simulink model "BMS"  (R2025b)
settings: Solver=VariableStepAuto  StartTime=0.0  StopTime=100000  RelTol=1e-3
libraries: fl_lib x15, nesl_utility x15, ee_lib x6, batteryecm_lib x5
settings DebuggingCC: AlgebraicLoopMsg=none

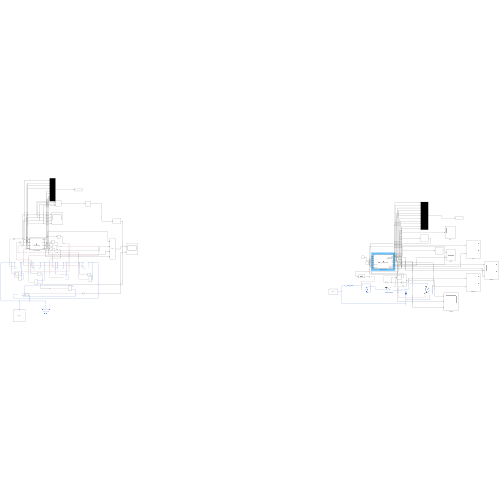
[thumbnail: Simulink's stored preview of the top-level diagram]
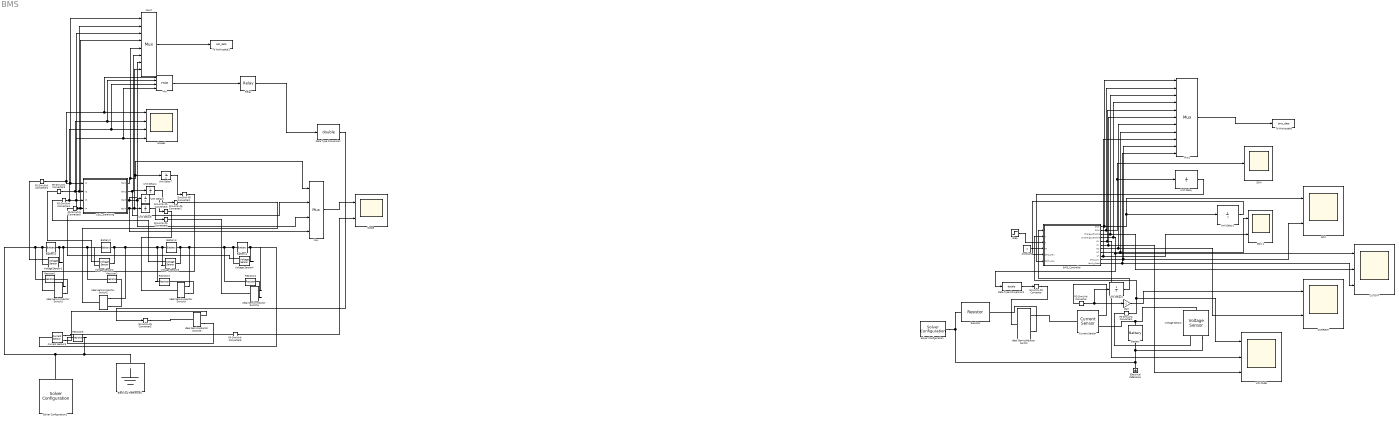
== system BMS ==
  BMS_Controller : MATLAB Function  TreatAsAtomicUnit=on
  Battery : batteryecm_lib/Battery  Vnom=48 V  prm_dir=simscape.enum.battery.prm_dir.disabled  R1_dis=2 Ohm  R1_ch=2 Ohm  R1=0.02 Ohm  prm_AH=simscape.enum.battery.prm_AH.finite  AH=50 A*hr  V1=46 V  AH1=40 A*hr  prm_R2=simscape.enum.battery.prm_R2.disabled  R2=2000 Ohm  Tmeas=298.15 K  charge_measurement_port=simscape.enum.battery.enable.no  prm_dyn=simscape.enum.battery.prm_dyn.off  Rp1=0.005 Ohm  tau1=30 s  Rp2=0.005 Ohm  tau2=30 s  Rp3=0.005 Ohm  tau3=30 s  Rp4=0.005 Ohm  tau4=30 s  Rp5=0.005 Ohm  tau5=30 s  prm_fade=simscape.enum.battery.prm_fade.disabled  N_fade=100  AH_fade=45 A*hr  R1_fade=2.02 Ohm  R1_ch_fade=2.02 Ohm  V1_fade=10.35 V  prm_age=simscape.enum.battery.prm_age.disabled  prm_age_OCV=simscape.enum.battery.prm_age_OCV.OCV  OCV_age=0.9  SOC_age=60  Tmeas_age=298.15 K  delta_time_age_vec=[0] d  temperature_age_vec=[273] K  OCV_scaling_age=2.2134e6  OCV_offset_age=1.632e6  temp_exp_age=0.515833569 V  t_exp_age=0.75  Vnom_T2=12 V  R1_T2=2.2 Ohm  R1_T2_dis=2.2 Ohm  R1_T2_ch=2.2 Ohm  V1_T2=11.4 V  R2_T2=2200 Ohm  Rp1_T2=0.005 Ohm  tau1_T2=30 s  Rp2_T2=0.005 Ohm  tau2_T2=30 s  Rp3_T2=0.005 Ohm  tau3_T2=30 s  Rp4_T2=0.005 Ohm  tau4_T2=30 s  Rp5_T2=0.005 Ohm  tau5_T2=30 s  Tmeas2=273.15 K  thermal_port=simscape.enum.thermaleffects.omit  thermal_mass=30000 J/K  i_specify=off  i_priority=None  i=0 A  i_nominal_specify=off  i_nominal_value=1  i_nominal_unit=A  v_specify=off  v_priority=None  v=0 V  v_nominal_specify=off  v_nominal_value=1  v_nominal_unit=V  charge_specify=off  charge_priority=High  charge=50 A*hr  charge_nominal_specify=off  charge_nominal_value=1  charge_nominal_unit=A*hr  num_cycles_specify=off  num_cycles_priority=High  num_cycles=0  num_cycles_nominal_specify=off  num_cycles_nominal_value=1  num_cycles_nominal_unit=1  temperature_specify=off  temperature_priority=High  temperature=298.15 K  temperature_nominal_specify=off  temperature_nominal_value=1  temperature_nominal_unit=K
  Battery1 : batteryecm_lib/Battery  Vnom=3.7 V  prm_dir=simscape.enum.battery.prm_dir.disabled  R1_dis=2 Ohm  R1_ch=2 Ohm  R1=0.02 Ohm  prm_AH=simscape.enum.battery.prm_AH.finite  AH=3 Ah  V1=3.45 V  AH1=2.7 Ah  prm_R2=simscape.enum.battery.prm_R2.disabled  R2=2000 Ohm  Tmeas=298.15 K  charge_measurement_port=simscape.enum.battery.enable.no  prm_dyn=simscape.enum.battery.prm_dyn.off  Rp1=0.005 Ohm  tau1=30 s  Rp2=0.005 Ohm  tau2=30 s  Rp3=0.005 Ohm  tau3=30 s  Rp4=0.005 Ohm  tau4=30 s  Rp5=0.005 Ohm  tau5=30 s  prm_fade=simscape.enum.battery.prm_fade.disabled  N_fade=100  AH_fade=45 A*hr  R1_fade=2.02 Ohm  R1_ch_fade=2.02 Ohm  V1_fade=10.35 V  prm_age=simscape.enum.battery.prm_age.disabled  prm_age_OCV=simscape.enum.battery.prm_age_OCV.OCV  OCV_age=0.9  SOC_age=60  Tmeas_age=298.15 K  delta_time_age_vec=[0] d  temperature_age_vec=[273] K  OCV_scaling_age=2.2134e6  OCV_offset_age=1.632e6  temp_exp_age=0.515833569 V  t_exp_age=0.75  Vnom_T2=12 V  R1_T2=2.2 Ohm  R1_T2_dis=2.2 Ohm  R1_T2_ch=2.2 Ohm  V1_T2=11.4 V  R2_T2=2200 Ohm  Rp1_T2=0.005 Ohm  tau1_T2=30 s  Rp2_T2=0.005 Ohm  tau2_T2=30 s  Rp3_T2=0.005 Ohm  tau3_T2=30 s  Rp4_T2=0.005 Ohm  tau4_T2=30 s  Rp5_T2=0.005 Ohm  tau5_T2=30 s  Tmeas2=273.15 K  thermal_port=simscape.enum.thermaleffects.omit  thermal_mass=30000 J/K  i_specify=off  i_priority=None  i=0 A  i_nominal_specify=off  i_nominal_value=1  i_nominal_unit=A  v_specify=off  v_priority=None  v=0 V  v_nominal_specify=off  v_nominal_value=1  v_nominal_unit=V  charge_specify=on  charge_priority=High  charge=2.7 Ah  charge_nominal_specify=off  charge_nominal_value=1  charge_nominal_unit=A*hr  num_cycles_specify=off  num_cycles_priority=High  num_cycles=0  num_cycles_nominal_specify=off  num_cycles_nominal_value=1  num_cycles_nominal_unit=1  temperature_specify=off  temperature_priority=High  temperature=298.15 K  temperature_nominal_specify=off  temperature_nominal_value=1  temperature_nominal_unit=K
  Battery2 : batteryecm_lib/Battery  Vnom=3.7 V  prm_dir=simscape.enum.battery.prm_dir.disabled  R1_dis=2 Ohm  R1_ch=2 Ohm  R1=0.02 Ohm  prm_AH=simscape.enum.battery.prm_AH.finite  AH=3 Ah  V1=3.35 V  AH1=2.4 Ah  prm_R2=simscape.enum.battery.prm_R2.disabled  R2=2000 Ohm  Tmeas=298.15 K  charge_measurement_port=simscape.enum.battery.enable.no  prm_dyn=simscape.enum.battery.prm_dyn.off  Rp1=0.005 Ohm  tau1=30 s  Rp2=0.005 Ohm  tau2=30 s  Rp3=0.005 Ohm  tau3=30 s  Rp4=0.005 Ohm  tau4=30 s  Rp5=0.005 Ohm  tau5=30 s  prm_fade=simscape.enum.battery.prm_fade.disabled  N_fade=100  AH_fade=45 A*hr  R1_fade=2.02 Ohm  R1_ch_fade=2.02 Ohm  V1_fade=10.35 V  prm_age=simscape.enum.battery.prm_age.disabled  prm_age_OCV=simscape.enum.battery.prm_age_OCV.OCV  OCV_age=0.9  SOC_age=60  Tmeas_age=298.15 K  delta_time_age_vec=[0] d  temperature_age_vec=[273] K  OCV_scaling_age=2.2134e6  OCV_offset_age=1.632e6  temp_exp_age=0.515833569 V  t_exp_age=0.75  Vnom_T2=12 V  R1_T2=2.2 Ohm  R1_T2_dis=2.2 Ohm  R1_T2_ch=2.2 Ohm  V1_T2=11.4 V  R2_T2=2200 Ohm  Rp1_T2=0.005 Ohm  tau1_T2=30 s  Rp2_T2=0.005 Ohm  tau2_T2=30 s  Rp3_T2=0.005 Ohm  tau3_T2=30 s  Rp4_T2=0.005 Ohm  tau4_T2=30 s  Rp5_T2=0.005 Ohm  tau5_T2=30 s  Tmeas2=273.15 K  thermal_port=simscape.enum.thermaleffects.omit  thermal_mass=30000 J/K  i_specify=off  i_priority=None  i=0 A  i_nominal_specify=off  i_nominal_value=1  i_nominal_unit=A  v_specify=off  v_priority=None  v=0 V  v_nominal_specify=off  v_nominal_value=1  v_nominal_unit=V  charge_specify=on  charge_priority=High  charge=2.4 Ah  charge_nominal_specify=off  charge_nominal_value=1  charge_nominal_unit=A*hr  num_cycles_specify=off  num_cycles_priority=High  num_cycles=0  num_cycles_nominal_specify=off  num_cycles_nominal_value=1  num_cycles_nominal_unit=1  temperature_specify=off  temperature_priority=High  temperature=298.15 K  temperature_nominal_specify=off  temperature_nominal_value=1  temperature_nominal_unit=K
  Battery3 : batteryecm_lib/Battery  Vnom=3.7 V  prm_dir=simscape.enum.battery.prm_dir.disabled  R1_dis=2 Ohm  R1_ch=2 Ohm  R1=0.02 Ohm  prm_AH=simscape.enum.battery.prm_AH.finite  AH=3 Ah  V1=3.25 V  AH1=2.1 Ah  prm_R2=simscape.enum.battery.prm_R2.disabled  R2=2000 Ohm  Tmeas=298.15 K  charge_measurement_port=simscape.enum.battery.enable.no  prm_dyn=simscape.enum.battery.prm_dyn.off  Rp1=0.005 Ohm  tau1=30 s  Rp2=0.005 Ohm  tau2=30 s  Rp3=0.005 Ohm  tau3=30 s  Rp4=0.005 Ohm  tau4=30 s  Rp5=0.005 Ohm  tau5=30 s  prm_fade=simscape.enum.battery.prm_fade.disabled  N_fade=100  AH_fade=45 A*hr  R1_fade=2.02 Ohm  R1_ch_fade=2.02 Ohm  V1_fade=10.35 V  prm_age=simscape.enum.battery.prm_age.disabled  prm_age_OCV=simscape.enum.battery.prm_age_OCV.OCV  OCV_age=0.9  SOC_age=60  Tmeas_age=298.15 K  delta_time_age_vec=[0] d  temperature_age_vec=[273] K  OCV_scaling_age=2.2134e6  OCV_offset_age=1.632e6  temp_exp_age=0.515833569 V  t_exp_age=0.75  Vnom_T2=12 V  R1_T2=2.2 Ohm  R1_T2_dis=2.2 Ohm  R1_T2_ch=2.2 Ohm  V1_T2=11.4 V  R2_T2=2200 Ohm  Rp1_T2=0.005 Ohm  tau1_T2=30 s  Rp2_T2=0.005 Ohm  tau2_T2=30 s  Rp3_T2=0.005 Ohm  tau3_T2=30 s  Rp4_T2=0.005 Ohm  tau4_T2=30 s  Rp5_T2=0.005 Ohm  tau5_T2=30 s  Tmeas2=273.15 K  thermal_port=simscape.enum.thermaleffects.omit  thermal_mass=30000 J/K  i_specify=off  i_priority=None  i=0 A  i_nominal_specify=off  i_nominal_value=1  i_nominal_unit=A  v_specify=off  v_priority=None  v=0 V  v_nominal_specify=off  v_nominal_value=1  v_nominal_unit=V  charge_specify=on  charge_priority=High  charge=2.1 Ah  charge_nominal_specify=off  charge_nominal_value=1  charge_nominal_unit=A*hr  num_cycles_specify=off  num_cycles_priority=High  num_cycles=0  num_cycles_nominal_specify=off  num_cycles_nominal_value=1  num_cycles_nominal_unit=1  temperature_specify=off  temperature_priority=High  temperature=298.15 K  temperature_nominal_specify=off  temperature_nominal_value=1  temperature_nominal_unit=K
  Battery4 : batteryecm_lib/Battery  Vnom=3.7 V  prm_dir=simscape.enum.battery.prm_dir.disabled  R1_dis=2 Ohm  R1_ch=2 Ohm  R1=0.02 Ohm  prm_AH=simscape.enum.battery.prm_AH.finite  AH=3 Ah  V1=3.15 V  AH1=1.8 Ah  prm_R2=simscape.enum.battery.prm_R2.disabled  R2=2000 Ohm  Tmeas=298.15 K  charge_measurement_port=simscape.enum.battery.enable.no  prm_dyn=simscape.enum.battery.prm_dyn.off  Rp1=0.005 Ohm  tau1=30 s  Rp2=0.005 Ohm  tau2=30 s  Rp3=0.005 Ohm  tau3=30 s  Rp4=0.005 Ohm  tau4=30 s  Rp5=0.005 Ohm  tau5=30 s  prm_fade=simscape.enum.battery.prm_fade.disabled  N_fade=100  AH_fade=45 A*hr  R1_fade=2.02 Ohm  R1_ch_fade=2.02 Ohm  V1_fade=10.35 V  prm_age=simscape.enum.battery.prm_age.disabled  prm_age_OCV=simscape.enum.battery.prm_age_OCV.OCV  OCV_age=0.9  SOC_age=60  Tmeas_age=298.15 K  delta_time_age_vec=[0] d  temperature_age_vec=[273] K  OCV_scaling_age=2.2134e6  OCV_offset_age=1.632e6  temp_exp_age=0.515833569 V  t_exp_age=0.75  Vnom_T2=12 V  R1_T2=2.2 Ohm  R1_T2_dis=2.2 Ohm  R1_T2_ch=2.2 Ohm  V1_T2=11.4 V  R2_T2=2200 Ohm  Rp1_T2=0.005 Ohm  tau1_T2=30 s  Rp2_T2=0.005 Ohm  tau2_T2=30 s  Rp3_T2=0.005 Ohm  tau3_T2=30 s  Rp4_T2=0.005 Ohm  tau4_T2=30 s  Rp5_T2=0.005 Ohm  tau5_T2=30 s  Tmeas2=273.15 K  thermal_port=simscape.enum.thermaleffects.omit  thermal_mass=30000 J/K  i_specify=off  i_priority=None  i=0 A  i_nominal_specify=off  i_nominal_value=1  i_nominal_unit=A  v_specify=off  v_priority=None  v=0 V  v_nominal_specify=off  v_nominal_value=1  v_nominal_unit=V  charge_specify=on  charge_priority=High  charge=1.8 Ah  charge_nominal_specify=off  charge_nominal_value=1  charge_nominal_unit=A*hr  num_cycles_specify=off  num_cycles_priority=High  num_cycles=0  num_cycles_nominal_specify=off  num_cycles_nominal_value=1  num_cycles_nominal_unit=1  temperature_specify=off  temperature_priority=High  temperature=298.15 K  temperature_nominal_specify=off  temperature_nominal_value=1  temperature_nominal_unit=K
  CELL_Balancing : MATLAB Function  TreatAsAtomicUnit=on
  CURRENT : Scope  NumInputPorts=2
      settings: ActiveDisplayYMinimum=-24.113371295047806  ActiveDisplayYMaximum=65.015748640986715
  CUTOFF : Scope  NumInputPorts=3
      settings: ActiveDisplayString=3  ActiveDisplayYMinimum=-1  ActiveDisplayYMaximum=7  DataLoggingVariableName=ScopeData2
  Constant : Constant
  Current Sensor : fl_lib/Electrical/Electrical Sensors/Current Sensor
  Current Sensor3 : fl_lib/Electrical/Electrical Sensors/Current Sensor
  Data Type Conversion : DataTypeConversion  OutDataTypeStr=double  SaturateOnIntegerOverflow=off  RndMeth=Floor
  Data Type Conversion1 : DataTypeConversion  OutDataTypeStr=double  SaturateOnIntegerOverflow=off  RndMeth=Floor
  Electrical Reference : fl_lib/Electrical/Electrical Elements/Electrical Reference
  Electrical Reference1 : fl_lib/Electrical/Electrical Elements/Electrical Reference
  Gain : Gain  Gain=-1
  Ideal Semiconductor Switch : ee_lib/Semiconductors & Converters/Ideal Semiconductor Switch  port_option=ee.enum.controlport.ps  Ron=0.001 Ohm  Goff=1e-6 1/Ohm  Vth=0.5 V  diode_param=ee.enum.semiconductors.protectionDiode.nodynamics  diode_Vf=0.8 V  diode_Ron=0.001 Ohm  diode_Goff=1e-5 1/Ohm  diode_C=50e-9 F  diode_iRM=-235 A  diode_iF=300 A  diode_idot=-50 A/us  diode_trr_param=ee.enum.converters.diodetrr.trr_factor  diode_trr_factor=3  diode_trr=15 us  diode_Qrr=1500 s*uA
  Ideal Semiconductor Switch{1..5} (5 alike) : ee_lib/Semiconductors & Converters/Ideal Semiconductor Switch  port_option=ee.enum.controlport.ps  Ron=0.1 Ohm  Goff=1e-6 S  Vth=0.5 V  diode_param=ee.enum.semiconductors.protectionDiode.external  diode_Vf=0.8 V  diode_Ron=0.001 Ohm  diode_Goff=1e-5 1/Ohm  diode_C=50e-9 F  diode_iRM=-235 A  diode_iF=300 A  diode_idot=-50 A/us  diode_trr_param=ee.enum.converters.diodetrr.trr_factor  diode_trr_factor=3  diode_trr=15 us  diode_Qrr=1500 s*uA
  Min : MinMax  Inputs=4
  Mux : Mux
  Mux1 : Mux  Inputs=11
  Mux2 : Mux  Inputs=8
  PS-Simulink Converter{,1..6} (7 alike) : nesl_utility/PS-Simulink Converter  PhysicalDomain=network_engine_domain  SubClassName=ps_output  LeftPortType=input  RightPortType=output  PseudoPeriodic=off  Frequencies=[]  VectorFormat=inherit  Unit=inherit  AffineConversion=off
  Relay : Relay  OnSwitchValue=3.0  OffSwitchValue=2.8
  Resistor : fl_lib/Electrical/Electrical Elements/Resistor  R=10 Ohm  i_specify=off  i_priority=None  i=0 A  i_nominal_specify=off  i_nominal_value=1  i_nominal_unit=A  v_specify=off  v_priority=None  v=0 V  v_nominal_specify=off  v_nominal_value=1  v_nominal_unit=V
  Resistor{1..4} (4 alike) : fl_lib/Electrical/Electrical Elements/Resistor  R=100 Ohm  i_specify=off  i_priority=None  i=0 A  i_nominal_specify=off  i_nominal_value=1  i_nominal_unit=A  v_specify=off  v_priority=None  v=0 V  v_nominal_specify=off  v_nominal_value=1  v_nominal_unit=V
  Resistor5 : fl_lib/Electrical/Electrical Elements/Resistor  R=50 Ohm  i_specify=off  i_priority=None  i=0 A  i_nominal_specify=off  i_nominal_value=1  i_nominal_unit=A  v_specify=off  v_priority=None  v=0 V  v_nominal_specify=off  v_nominal_value=1  v_nominal_unit=V
  "SOC " : Scope  NumInputPorts=2
      settings: ActiveDisplayYMinimum=0  ActiveDisplayYMaximum=1.05
  SOC 1 : Scope  NumInputPorts=2
      settings: ActiveDisplayYMinimum=-1  ActiveDisplayYMaximum=2  DataLoggingVariableName=ScopeData7
  SOH : Scope
      settings: ActiveDisplayYMinimum=0.7  ActiveDisplayYMaximum=1.01  DataLoggingVariableName=ScopeData4
  Scope : Scope  NumInputPorts=2
      settings: ActiveDisplayYMinimum=-0.08125912986411854  ActiveDisplayYMaximum=1.0773261926772566  DataLoggingVariableName=ScopeData5
  Scope1 : Scope  NumInputPorts=4
      settings: ActiveDisplayString=4  ActiveDisplayYMinimum=2  ActiveDisplayYMaximum=5  DataLoggingVariableName=ScopeData6
  Simulink-PS Converter{,1..5} (6 alike) : nesl_utility/Simulink-PS Converter  PhysicalDomain=network_engine_domain  SubClassName=ps_input  LeftPortType=input  RightPortType=output  PseudoPeriodic=off  Frequencies=[]  NoiseDistribution=none  NoiseParameters=[]  Unit=1  AffineConversion=off  FilteringAndDerivatives=provide  SimscapeFilterOrder=1  InputFilterTimeConstant=0.001  UdotUserProvided=0
  Solver Configuration : nesl_utility/Solver Configuration  PhysicalDomain=network_engine_domain  SubClassName=solver  LeftPortType=input  RightPortType=generic  Tones=[]  Harmonics=[]  SimulateNoise=off  Profile=off  UseLocalSampling=off  EnableSwitchedLinearOptims=on  FrequencyDomain=off  UseCCode=off  RelTol=0.001  AbsTol=0.001  MinStep=1e-09  ToWorkspace=off  RevertToSquareIcSolve=off  NumHomotopyIterations=100  PhasorMode=off  PhasorModeNumHarmonics=1  ConsistencySolver=NEWTON_XTOL_AFTER_FTOL  IndexReductionMethod=DerivativeReplacement  DoDC=off  ResidualTolerance=1e-09  ConsistencyTolSource=GLOBAL  ConsistencyAbsTol=0.001  ConsistencyRelTol=0.001  ConsistencyTolFactor=0.001  UseLocalSolver=off  LocalSolverChoice=NE_BACKWARD_EULER_ADVANCER  ResolveIndetEquations=on  FunctionEvalNumThread=1  LocalSolverSampleTime=0.001  DoFixedCost=off  MaxNonlinIter=3  MaxModeIter=2  ComputeImpulses=off  ImpulseIterations=2  LinearAlgebra=auto  LinearAlgebraNumThread=0  EquationFormulation=NE_TIME_EF  DelaysMemoryBudget=1024  AutomaticFiltering=on  FilteringTimeConstant=0.001  PartitionStorageMethod=AS_NEEDED  PartitionMemoryBudget=1024  PartitionMethod=ROBUST  MultibodyUseLocalSolver=off  MultibodyLocalSolverChoice=ODE1  MultibodyLocalSolverSampleTime=0.001
  Solver Configuration1 : nesl_utility/Solver Configuration  PhysicalDomain=network_engine_domain  SubClassName=solver  LeftPortType=input  RightPortType=generic  Tones=[]  Harmonics=[]  SimulateNoise=off  Profile=off  UseLocalSampling=off  EnableSwitchedLinearOptims=on  FrequencyDomain=off  UseCCode=off  RelTol=0.001  AbsTol=0.001  MinStep=1e-09  ToWorkspace=off  RevertToSquareIcSolve=off  NumHomotopyIterations=100  PhasorMode=off  PhasorModeNumHarmonics=1  ConsistencySolver=NEWTON_XTOL_AFTER_FTOL  IndexReductionMethod=DerivativeReplacement  DoDC=off  ResidualTolerance=1e-09  ConsistencyTolSource=GLOBAL  ConsistencyAbsTol=0.001  ConsistencyRelTol=0.001  ConsistencyTolFactor=0.001  UseLocalSolver=off  LocalSolverChoice=NE_BACKWARD_EULER_ADVANCER  ResolveIndetEquations=on  FunctionEvalNumThread=1  LocalSolverSampleTime=0.001  DoFixedCost=off  MaxNonlinIter=3  MaxModeIter=2  ComputeImpulses=off  ImpulseIterations=2  LinearAlgebra=auto  LinearAlgebraNumThread=0  EquationFormulation=NE_TIME_EF  DelaysMemoryBudget=1024  AutomaticFiltering=on  FilteringTimeConstant=0.001  PartitionStorageMethod=AS_NEEDED  PartitionMemoryBudget=1024  PartitionMethod=ROBUST  MultibodyUseLocalSolver=off  MultibodyLocalSolverChoice=ODE1  MultibodyLocalSolverSampleTime=0.001
  Step : Step  Time=5000  Before=25  After=70  SampleTime=0
  To Workspace : ToWorkspace  VariableName=bms_data  SaveFormat=Structure With Time  SampleTime=-1
  To Workspace1 : ToWorkspace  VariableName=cell_data  SaveFormat=Structure With Time  SampleTime=-1
  Unit Delay : UnitDelay  InitialCondition=1  HasFrameUpgradeWarning=on
  Unit Delay1 : UnitDelay  InitialCondition=1  HasFrameUpgradeWarning=on
  Unit Delay2 : UnitDelay  HasFrameUpgradeWarning=on
  Unit Delay{4..7} (4 alike) : UnitDelay  SampleTime=-1  HasFrameUpgradeWarning=on
  VOLTAGE : Scope  NumInputPorts=3
      settings: ActiveDisplayString=3  ActiveDisplayYMinimum=-5  ActiveDisplayYMaximum=54  DataLoggingVariableName=ScopeData3
  Voltage Sensor{,1..4} (5 alike) : fl_lib/Electrical/Electrical Sensors/Voltage Sensor
  wires:
  PS-Simulink Converter/1 -> Unit Delay2/1, Gain/1
  PS-Simulink Converter1/1 -> BMS_Controller/2(V), VOLTAGE/1
  Constant/1 -> BMS_Controller/4(Ts)
  BMS_Controller/1(SOC) -> Mux1/1, "SOC "/1, Unit Delay1/1
  Unit Delay1/1 -> BMS_Controller/5(SOC_prev)
  Gain/1 -> CURRENT/1
  BMS_Controller/5(OV) -> Mux1/5, VOLTAGE/2
  BMS_Controller/2(SOH) -> Mux1/2, SOH/1, Unit Delay/1
  Unit Delay2/1 -> BMS_Controller/1(I)
  PS-Simulink Converter2/1 -> Min/1, Scope1/1, Mux2/1, CELL_Balancing/1(V1)
  PS-Simulink Converter3/1 -> Min/2, Scope1/2, CELL_Balancing/2(V2), Mux2/2
  PS-Simulink Converter4/1 -> Mux2/3, CELL_Balancing/3(V3), Min/3, Scope1/3
  CELL_Balancing/1(Bal1) -> Mux2/5, Unit Delay7/1, Mux/1
  CELL_Balancing/2(Bal2) -> Mux2/6, Unit Delay4/1, Mux/2
  CELL_Balancing/3(Bal3) -> Mux2/7, Unit Delay5/1, Mux/3
  Unit Delay7/1 -> Simulink-PS Converter1/1
  Unit Delay4/1 -> Simulink-PS Converter2/1
  Unit Delay5/1 -> Simulink-PS Converter3/1
  Unit Delay6/1 -> Simulink-PS Converter4/1
  Mux/1 -> Scope/1
  PS-Simulink Converter6/1 -> Scope/2
  Data Type Conversion/1 -> Simulink-PS Converter5/1
  CELL_Balancing/4(Bal4) -> Mux/4, Mux2/8, Unit Delay6/1
  Min/1 -> Relay/1
  Relay/1 -> Data Type Conversion/1
  Unit Delay/1 -> BMS_Controller/6(SOH_prev)
  Step/1 -> BMS_Controller/3(T)
  BMS_Controller/7(OC) -> Mux1/7, CURRENT/2
  BMS_Controller/10(SOC_Low) -> Mux1/10, "SOC "/2
  BMS_Controller/8(OT) -> Mux1/8, SOC 1/1
  BMS_Controller/9(UT) -> Mux1/9, SOC 1/2
  BMS_Controller/6(UV) -> Mux1/6, VOLTAGE/3
  BMS_Controller/4(Discharge_Enable) -> Mux1/4, Data Type Conversion1/1, CUTOFF/1
  Data Type Conversion1/1 -> Simulink-PS Converter/1
  BMS_Controller/3(Charge_Enable) -> Mux1/3, CUTOFF/2
  BMS_Controller/11(Fault_Code) -> Mux1/11, CUTOFF/3
  Mux1/1 -> To Workspace/1
  PS-Simulink Converter5/1 -> Mux2/4, CELL_Balancing/4(V4), Min/4, Scope1/4
  Mux2/1 -> To Workspace1/1
  connections:
  Battery/RConn1 -- Voltage Sensor/RConn2 -- Electrical Reference/LConn1 -- Solver Configuration/RConn1 -- Resistor/LConn1
  Battery/LConn1 -- Current Sensor/RConn2 -- Voltage Sensor/LConn1
  PS-Simulink Converter/LConn1 -- Current Sensor/RConn1
  PS-Simulink Converter1/LConn1 -- Voltage Sensor/RConn1
  Current Sensor/LConn1 -- Ideal Semiconductor Switch/RConn1
  Simulink-PS Converter/RConn1 -- Ideal Semiconductor Switch/LConn1
  Ideal Semiconductor Switch/RConn2 -- Resistor/RConn1
  PS-Simulink Converter2/LConn1 -- Voltage Sensor1/RConn1
  Voltage Sensor4/LConn1 -- Current Sensor3/LConn1 -- Ideal Semiconductor Switch4/RConn1 -- Battery4/LConn1
  PS-Simulink Converter5/LConn1 -- Voltage Sensor4/RConn1
  PS-Simulink Converter3/LConn1 -- Voltage Sensor2/RConn1
  PS-Simulink Converter4/LConn1 -- Voltage Sensor3/RConn1
  Ideal Semiconductor Switch1/RConn2 -- Resistor1/LConn1
  Ideal Semiconductor Switch2/RConn2 -- Resistor2/LConn1
  Ideal Semiconductor Switch3/RConn2 -- Resistor3/LConn1
  Ideal Semiconductor Switch4/RConn2 -- Resistor4/LConn1
  Simulink-PS Converter2/RConn1 -- Ideal Semiconductor Switch2/LConn1
  Simulink-PS Converter3/RConn1 -- Ideal Semiconductor Switch3/LConn1
  Simulink-PS Converter4/RConn1 -- Ideal Semiconductor Switch4/LConn1
  Voltage Sensor1/LConn1 -- Resistor2/RConn1 -- Voltage Sensor2/RConn2 -- Battery2/RConn1 -- Ideal Semiconductor Switch1/RConn1 -- Battery1/LConn1
  Voltage Sensor2/LConn1 -- Resistor3/RConn1 -- Voltage Sensor3/RConn2 -- Battery3/RConn1 -- Ideal Semiconductor Switch2/RConn1 -- Battery2/LConn1
  Voltage Sensor3/LConn1 -- Voltage Sensor4/RConn2 -- Battery4/RConn1 -- Resistor4/RConn1 -- Ideal Semiconductor Switch3/RConn1 -- Battery3/LConn1
  Current Sensor3/RConn1 -- PS-Simulink Converter6/LConn1
  Current Sensor3/RConn2 -- Ideal Semiconductor Switch5/RConn1
  Ideal Semiconductor Switch5/RConn2 -- Resistor5/LConn1
  Simulink-PS Converter5/RConn1 -- Ideal Semiconductor Switch5/LConn1
  Simulink-PS Converter1/RConn1 -- Ideal Semiconductor Switch1/LConn1
  Battery1/RConn1 -- Voltage Sensor1/RConn2 -- Resistor1/RConn1 -- Resistor5/RConn1 -- Electrical Reference1/LConn1 -- Solver Configuration1/RConn1

== matlab function BMS/CELL_Balancing ==
  data: V1 input; Bal1 output; V2 input; V3 input; V4 input; Bal2 output; Bal3 output; Bal4 output
function [Bal1, Bal2, Bal3, Bal4] = Cell_Balancing(V1, V2, V3, V4)

%#codegen

%% Initialize outputs
Bal1 = 0;
Bal2 = 0;
Bal3 = 0;
Bal4 = 0;

%% Threshold
DeltaV = 0.05;   % 50 mV

%% Maximum cell voltage
Vmax = max([V1, V2, V3, V4]);

%% Balancing logic
if V1 > (Vmax - DeltaV) && V1>2.8
    Bal1 = 1;
end

if V2 > (Vmax - DeltaV)  && V2>2.8
    Bal2 = 1;
end

if V3 > (Vmax - DeltaV)  && V3>2.8
    Bal3 = 1;
end

if V4 > (Vmax - DeltaV)  && V4>2.8
    Bal4 = 1;
end

end

== matlab function BMS/BMS_Controller ==
  settings: updateMethod=DISCRETE
  data: SOC output double size=1*1; SOH output; I input; V input; T input; Ts input; Charge_Enable output double size=1*1; Discharge_Enable output; OV output; SOC_prev input; SOH_prev input; UV output; OC output; OT output; UT output; SOC_Low output; Fault_Code output
function [SOC, SOH, Charge_Enable, Discharge_Enable, ...
          OV, UV, OC, OT, UT, SOC_Low, Fault_Code] = ...
    BMS_Controller_Day9(I, V, T, Ts, SOC_prev, SOH_prev)

%#codegen

%% Initialize outputs
SOC = SOC_prev;
SOH = SOH_prev;

Charge_Enable = 1;
Discharge_Enable = 1;

OV = 0; 
UV = 0; 
OC = 0; 
OT = 0; 
UT = 0; 
SOC_Low = 0;

Fault_Code = 0;

%% Parameters
C_nom = 50;          % Ah

SOC_cutoff = 0.2;
SOC_recover = 0.25;

V_min = 42;          % Pack voltage
V_max = 54;

I_max = 8;           % Max current

T_min = 0;           % °C
T_max = 60;

%% Separate charge and discharge current
if I >= 0
    I_dis = I;
    I_chg = 0;
else
    I_dis = 0;
    I_chg = -I;
end

%% SOC calculation
SOC = SOC_prev ...
    - (I_dis * Ts)/(3600*C_nom) ...
    + (I_chg * Ts)/(3600*C_nom);

SOC = max(0, min(1, SOC));

%% SOH degradation (very slow)
SOH = SOH_prev - (I_dis * Ts)/(3600*200000);
SOH = max(0.7, min(1, SOH));

%% Voltage faults
if V > V_max
    OV = 1;
end

if V < V_min
    UV = 1;
end

%% Current fault
if abs(I) > I_max
    OC = 1;
end

%% Temperature faults
if T > T_max
    OT = 1;
end

if T < T_min
    UT = 1;
end

%% SOC hysteresis
if SOC <= SOC_cutoff
    SOC_Low = 1;
elseif SOC >= SOC_recover
    SOC_Low = 0;
end

%% Discharge control logic
if (UV==1) || (OC==1) || (OT==1) || (SOC_Low==1)
    Discharge_Enable = 0;
end

%% Charge control logic
if (OV==1) || (OT==1) || (UT==1)
    Charge_Enable = 0;
end

%% Fault code assignment
% 0 = No fault
% 1 = Over Voltage
% 2 = Under Voltage
% 3 = Over Current
% 4 = Over Temp
% 5 = Under Temp
% 6 = Low SOC

if OV==1
    Fault_Code = 1;
elseif UV==1
    Fault_Code = 2;
elseif OC==1
    Fault_Code = 3;
elseif OT==1
    Fault_Code = 4;
elseif UT==1
    Fault_Code = 5;
elseif SOC_Low==1
    Fault_Code = 6;
end

end
